simulink model "calibration_jacobian_n_8"  (R2018b)
settings: Solver=VariableStepAuto  StartTime=0.0  StopTime=10  RelTol=1e-3
values from neighbouring files (symbols this model uses):
  base_size = [0.2 0.3 1.5]    [robot_setup.m]    (also in robot_setup_delta_l.m)
  beam_length = 1.14    [robot_setup.m]    (also in robot_setup_delta_l.m)
  beam_radius = 0.032    [robot_setup.m]    (also in robot_setup_delta_l.m)
  fixture_height = 1.5    [robot_setup.m]    (also in robot_setup_delta_l.m)
  robot_frame_x = 0.15    [robot_setup.m]    (also in robot_setup_delta_l.m)
  T = 0.005    [robot_setup.m]    (also in robot_setup_delta_l.m)
  theta_m_des_calib = 0    [robot_setup_delta_l.m]
  wf_T_rf_left = [R_left, xyz_left'; 0 0 0 1]    [robot_setup.m]    (also in robot_setup_delta_l.m)
  wf_T_rf_right = [R_right, xyz_right'; 0 0 0 1]    [robot_setup.m]    (also in robot_setup_delta_l.m)
  xyz_0_rf_left = xyz_0_rf_left(1:3)    [robot_setup.m]    (also in robot_setup_delta_l.m)
  xyz_0_rf_right = xyz_0_rf_right(1:3)    [robot_setup.m]    (also in robot_setup_delta_l.m)
  yd_des_calib = 1    [robot_setup.m]    (also in robot_setup_delta_l.m = 0.9)
  ym_des_calib = 0    [robot_setup.m]    (also in robot_setup_delta_l.m)
  zd_des_calib = 0    [robot_setup.m]    (also in robot_setup_delta_l.m)
  zm_des_calib = 1.5    [robot_setup.m]    (also in robot_setup_delta_l.m)
undefined symbols (not defined in the file or in its folder): beam_wall, beam_width, Extr_Data_Box, Levenberg, Marquardt, num_elements, X, Y, Z
libraries: sm_lib x349, nesl_utility x63, sm_flex_body_lib x12, robotcorelib x4, simulink x2, robotmaniplib x2
(part 8 of 8)

== system calibration_jacobian_n_8/KUKA IIWA right/KUKA_iiwa 1 /iiwa_link_6 ==
  Inertia : sm_lib/Body Elements/Inertia  InertiaType=Custom  Mass=2.3466  MassUnits=kg  CenterOfMass=[0, 0, 0]  CenterOfMassUnits=m  MomentsOfInertia=[0.006509, 0.006259, 0.004527]  MomentsOfInertiaUnits=kg*m^2  ProductsOfInertia=[0.00031891, 0, 0]  ProductsOfInertiaUnits=kg*m^2  GraphicType=None  MarkerShape=Inertia  MarkerSize=20  GraphicVisPropType=SimpleVisualProperties  GraphicDiffuseColor=[0.5 0.5 0.5]  GraphicSpecularColor=[0.5 0.5 0.5 1.0]  GraphicAmbientColor=[0.15 0.15 0.15 1.0]  GraphicEmissiveColor=[0.0 0.0 0.0 1.0]  GraphicShininess=75  GraphicOpacity=1.0
  InertiaOriginTransform : sm_lib/Frames and Transforms/Rigid Transform  TranslationMethod=Cartesian  TranslationStandardOffset=0  TranslationLengthUnit=m  TranslationStandardAxis=+Z  TranslationCartesianOffset=[0, 0.0005999999999999999, 0.0004]  TranslationROffset=0  TranslationROffsetUnits=m  TranslationZOffset=0  TranslationZOffsetUnits=m  TranslationThetaOffset=0  TranslationThetaOffsetUnits=deg  RotationMethod=RotationSequence  RotationAngleUnits=deg  RotationStandardAxis=+Z  RotationAngle=0.0  RotationArbitraryAxis=[0 0 1]  FollAlignAxisA=+X  BaseAlignAxisA=+Y  FollAlignAxisB=+Y  BaseAlignAxisB=+Z  RotationSequenceAxes=BaseAxes  RotationSequence=XYZ  RotationSequenceAngles=[0, 0, 0]  RotationSequenceAnglesUnits=rad  RotationMatrix=[1 0 0; 0 1 0; 0 0 1]
  ReferenceFrame : sm_lib/Frames and Transforms/Reference Frame
  Visual : sm_lib/Body Elements/Solid  InertiaType=Custom  Mass=0  MassUnits=kg  CenterOfMass=[0, 0, 0]  CenterOfMassUnits=m  MomentsOfInertia=[0, 0, 0]  MomentsOfInertiaUnits=kg*m^2  ProductsOfInertia=[0, 0, 0]  ProductsOfInertiaUnits=kg*m^2  BasedOnType=Density  Density=1000  DensityUnits=kg/m^3  DoExposeReferenceFrame=on  SerializedFrames=<Frames/>  GraphicType=FromGeometry  MarkerShape=Sphere  MarkerSize=10  GraphicVisPropType=SimpleVisualProperties  GraphicDiffuseColor=[1, 0.423529411765, 0.0392156862745]  GraphicSpecularColor=[0.5 0.5 0.5 1.0]  GraphicAmbientColor=[0.15 0.15 0.15 1.0]  GraphicEmissiveColor=[0.0 0.0 0.0 1.0]  GraphicShininess=75  GraphicOpacity=1  GeometryShape=FromFile  RectangleSize=[1 1]  RectangleSizeUnits=m  BrickDimensions=[1 1 1]  BrickDimensionUnits=m  CylinderRadius=1  CylinderRadiusUnits=m  CylinderLength=1  CylinderLengthUnits=m  SphereRadius=1  SphereRadiusUnits=m  EllipsoidRadii=[1 1 1]  EllipsoidRadiiUnits=m  ExtrusionCrossSection=[1 1; -1 1; -1 -1; 1 -1]  ExtrusionCrossSectionUnits=m  ExtrusionLength=1  ExtrusionLengthUnits=m  PolygonNumSides=3  PolygonOuterRadius=1  PolygonOuterRadiusUnits=m  ExtGeomFileType=STL  ExtGeomFileName=iiwa_description/meshes/iiwa7/visual/link_6.stl  ExtGeomFileUnits=m  RevolutionCrossSection=[1 1; 1 -1; 2 -1; 2 1]  RevolutionCrossSectionUnits=m  RevolutionExtent=Full  RevolutionAngle=180  RevolutionAngleUnits=deg
  VisualOriginTransform : sm_lib/Frames and Transforms/Rigid Transform  TranslationMethod=Cartesian  TranslationStandardOffset=0  TranslationLengthUnit=m  TranslationStandardAxis=+Z  TranslationCartesianOffset=[0, 0, 0]  TranslationROffset=0  TranslationROffsetUnits=m  TranslationZOffset=0  TranslationZOffsetUnits=m  TranslationThetaOffset=0  TranslationThetaOffsetUnits=deg  RotationMethod=RotationSequence  RotationAngleUnits=deg  RotationStandardAxis=+Z  RotationAngle=0.0  RotationArbitraryAxis=[0 0 1]  FollAlignAxisA=+X  BaseAlignAxisA=+Y  FollAlignAxisB=+Y  BaseAlignAxisB=+Z  RotationSequenceAxes=BaseAxes  RotationSequence=XYZ  RotationSequenceAngles=[0, 0, 0]  RotationSequenceAnglesUnits=rad  RotationMatrix=[1 0 0; 0 1 0; 0 0 1]
  iiwa_joint_6_AxisInvTransform : sm_lib/Frames and Transforms/Rigid Transform  TranslationMethod=Cartesian  TranslationStandardOffset=0  TranslationLengthUnit=m  TranslationStandardAxis=+Z  TranslationCartesianOffset=[0, 0, 0]  TranslationROffset=0  TranslationROffsetUnits=m  TranslationZOffset=0  TranslationZOffsetUnits=m  TranslationThetaOffset=0  TranslationThetaOffsetUnits=deg  RotationMethod=ArbitraryAxis  RotationAngleUnits=rad  RotationStandardAxis=+Z  RotationAngle=0  RotationArbitraryAxis=[1, 0, 0]  FollAlignAxisA=+X  BaseAlignAxisA=+Y  FollAlignAxisB=+Y  BaseAlignAxisB=+Z  RotationSequenceAxes=FollowerAxes  RotationSequence=XYX  RotationSequenceAngles=[0 0 0]  RotationSequenceAnglesUnits=deg  RotationMatrix=[1 0 0; 0 1 0; 0 0 1]
  iiwa_joint_7_AxisTransform : sm_lib/Frames and Transforms/Rigid Transform  TranslationMethod=Cartesian  TranslationStandardOffset=0  TranslationLengthUnit=m  TranslationStandardAxis=+Z  TranslationCartesianOffset=[0, 0, 0]  TranslationROffset=0  TranslationROffsetUnits=m  TranslationZOffset=0  TranslationZOffsetUnits=m  TranslationThetaOffset=0  TranslationThetaOffsetUnits=deg  RotationMethod=ArbitraryAxis  RotationAngleUnits=rad  RotationStandardAxis=+Z  RotationAngle=0  RotationArbitraryAxis=[1, 0, 0]  FollAlignAxisA=+X  BaseAlignAxisA=+Y  FollAlignAxisB=+Y  BaseAlignAxisB=+Z  RotationSequenceAxes=FollowerAxes  RotationSequence=XYX  RotationSequenceAngles=[0 0 0]  RotationSequenceAnglesUnits=deg  RotationMatrix=[1 0 0; 0 1 0; 0 0 1]
  iiwa_joint_7_OriginTransform : sm_lib/Frames and Transforms/Rigid Transform  TranslationMethod=Cartesian  TranslationStandardOffset=0  TranslationLengthUnit=m  TranslationStandardAxis=+Z  TranslationCartesianOffset=[0, 0.081, 0.0607]  TranslationROffset=0  TranslationROffsetUnits=m  TranslationZOffset=0  TranslationZOffsetUnits=m  TranslationThetaOffset=0  TranslationThetaOffsetUnits=deg  RotationMethod=RotationSequence  RotationAngleUnits=deg  RotationStandardAxis=+Z  RotationAngle=0.0  RotationArbitraryAxis=[0 0 1]  FollAlignAxisA=+X  BaseAlignAxisA=+Y  FollAlignAxisB=+Y  BaseAlignAxisB=+Z  RotationSequenceAxes=BaseAxes  RotationSequence=XYZ  RotationSequenceAngles=[-1.57079632679, 3.14159265359, 0]  RotationSequenceAnglesUnits=rad  RotationMatrix=[1 0 0; 0 1 0; 0 0 1]
  F : PMIOPort  Side=Left
  F1 : PMIOPort  Port=2  Side=Right
  connections:
  Inertia/RConn1 -- InertiaOriginTransform/RConn1
  ReferenceFrame/RConn1 -- InertiaOriginTransform/LConn1 -- VisualOriginTransform/LConn1 -- iiwa_joint_6_AxisInvTransform/LConn1 -- iiwa_joint_7_OriginTransform/LConn1
  Visual/RConn1 -- VisualOriginTransform/RConn1
  iiwa_joint_6_AxisInvTransform/RConn1 -- F/RConn1
  iiwa_joint_7_AxisTransform/RConn1 -- F1/RConn1
  iiwa_joint_7_AxisTransform/LConn1 -- iiwa_joint_7_OriginTransform/RConn1

== system calibration_jacobian_n_8/KUKA IIWA right/KUKA_iiwa 1 /iiwa_link_7 ==
  Inertia : sm_lib/Body Elements/Inertia  InertiaType=Custom  Mass=3.129  MassUnits=kg  CenterOfMass=[0, 0, 0]  CenterOfMassUnits=m  MomentsOfInertia=[0.01464, 0.01465, 0.002872]  MomentsOfInertiaUnits=kg*m^2  ProductsOfInertia=[0, 0, 0.0005912]  ProductsOfInertiaUnits=kg*m^2  GraphicType=None  MarkerShape=Inertia  MarkerSize=20  GraphicVisPropType=SimpleVisualProperties  GraphicDiffuseColor=[0.5 0.5 0.5]  GraphicSpecularColor=[0.5 0.5 0.5 1.0]  GraphicAmbientColor=[0.15 0.15 0.15 1.0]  GraphicEmissiveColor=[0.0 0.0 0.0 1.0]  GraphicShininess=75  GraphicOpacity=1.0
  InertiaOriginTransform : sm_lib/Frames and Transforms/Rigid Transform  TranslationMethod=Cartesian  TranslationStandardOffset=0  TranslationLengthUnit=m  TranslationStandardAxis=+Z  TranslationCartesianOffset=[0, 0, 0.02]  TranslationROffset=0  TranslationROffsetUnits=m  TranslationZOffset=0  TranslationZOffsetUnits=m  TranslationThetaOffset=0  TranslationThetaOffsetUnits=deg  RotationMethod=RotationSequence  RotationAngleUnits=deg  RotationStandardAxis=+Z  RotationAngle=0.0  RotationArbitraryAxis=[0 0 1]  FollAlignAxisA=+X  BaseAlignAxisA=+Y  FollAlignAxisB=+Y  BaseAlignAxisB=+Z  RotationSequenceAxes=BaseAxes  RotationSequence=XYZ  RotationSequenceAngles=[0, 0, 0]  RotationSequenceAnglesUnits=rad  RotationMatrix=[1 0 0; 0 1 0; 0 0 1]
  ReferenceFrame : sm_lib/Frames and Transforms/Reference Frame
  Visual : sm_lib/Body Elements/Solid  InertiaType=Custom  Mass=0  MassUnits=kg  CenterOfMass=[0, 0, 0]  CenterOfMassUnits=m  MomentsOfInertia=[0, 0, 0]  MomentsOfInertiaUnits=kg*m^2  ProductsOfInertia=[0, 0, 0]  ProductsOfInertiaUnits=kg*m^2  BasedOnType=Density  Density=1000  DensityUnits=kg/m^3  DoExposeReferenceFrame=on  SerializedFrames=<Frames/>  GraphicType=FromGeometry  MarkerShape=Sphere  MarkerSize=10  GraphicVisPropType=SimpleVisualProperties  GraphicDiffuseColor=[0.4, 0.4, 0.4]  GraphicSpecularColor=[0.5 0.5 0.5 1.0]  GraphicAmbientColor=[0.15 0.15 0.15 1.0]  GraphicEmissiveColor=[0.0 0.0 0.0 1.0]  GraphicShininess=75  GraphicOpacity=1  GeometryShape=FromFile  RectangleSize=[1 1]  RectangleSizeUnits=m  BrickDimensions=[1 1 1]  BrickDimensionUnits=m  CylinderRadius=1  CylinderRadiusUnits=m  CylinderLength=1  CylinderLengthUnits=m  SphereRadius=1  SphereRadiusUnits=m  EllipsoidRadii=[1 1 1]  EllipsoidRadiiUnits=m  ExtrusionCrossSection=[1 1; -1 1; -1 -1; 1 -1]  ExtrusionCrossSectionUnits=m  ExtrusionLength=1  ExtrusionLengthUnits=m  PolygonNumSides=3  PolygonOuterRadius=1  PolygonOuterRadiusUnits=m  ExtGeomFileType=STL  ExtGeomFileName=iiwa_description/meshes/iiwa7/visual/link_7.stl  ExtGeomFileUnits=m  RevolutionCrossSection=[1 1; 1 -1; 2 -1; 2 1]  RevolutionCrossSectionUnits=m  RevolutionExtent=Full  RevolutionAngle=180  RevolutionAngleUnits=deg
  VisualOriginTransform : sm_lib/Frames and Transforms/Rigid Transform  TranslationMethod=Cartesian  TranslationStandardOffset=0  TranslationLengthUnit=m  TranslationStandardAxis=+Z  TranslationCartesianOffset=[0, 0, -0.0005]  TranslationROffset=0  TranslationROffsetUnits=m  TranslationZOffset=0  TranslationZOffsetUnits=m  TranslationThetaOffset=0  TranslationThetaOffsetUnits=deg  RotationMethod=RotationSequence  RotationAngleUnits=deg  RotationStandardAxis=+Z  RotationAngle=0.0  RotationArbitraryAxis=[0 0 1]  FollAlignAxisA=+X  BaseAlignAxisA=+Y  FollAlignAxisB=+Y  BaseAlignAxisB=+Z  RotationSequenceAxes=BaseAxes  RotationSequence=XYZ  RotationSequenceAngles=[0, 0, 0]  RotationSequenceAnglesUnits=rad  RotationMatrix=[1 0 0; 0 1 0; 0 0 1]
  iiwa_joint_7_AxisInvTransform : sm_lib/Frames and Transforms/Rigid Transform  TranslationMethod=Cartesian  TranslationStandardOffset=0  TranslationLengthUnit=m  TranslationStandardAxis=+Z  TranslationCartesianOffset=[0, 0, 0]  TranslationROffset=0  TranslationROffsetUnits=m  TranslationZOffset=0  TranslationZOffsetUnits=m  TranslationThetaOffset=0  TranslationThetaOffsetUnits=deg  RotationMethod=ArbitraryAxis  RotationAngleUnits=rad  RotationStandardAxis=+Z  RotationAngle=0  RotationArbitraryAxis=[1, 0, 0]  FollAlignAxisA=+X  BaseAlignAxisA=+Y  FollAlignAxisB=+Y  BaseAlignAxisB=+Z  RotationSequenceAxes=FollowerAxes  RotationSequence=XYX  RotationSequenceAngles=[0 0 0]  RotationSequenceAnglesUnits=deg  RotationMatrix=[1 0 0; 0 1 0; 0 0 1]
  iiwa_joint_ee_OriginTransform : sm_lib/Frames and Transforms/Rigid Transform  TranslationMethod=Cartesian  TranslationStandardOffset=0  TranslationLengthUnit=m  TranslationStandardAxis=+Z  TranslationCartesianOffset=[0, 0, 0.045]  TranslationROffset=0  TranslationROffsetUnits=m  TranslationZOffset=0  TranslationZOffsetUnits=m  TranslationThetaOffset=0  TranslationThetaOffsetUnits=deg  RotationMethod=RotationSequence  RotationAngleUnits=deg  RotationStandardAxis=+Z  RotationAngle=0.0  RotationArbitraryAxis=[0 0 1]  FollAlignAxisA=+X  BaseAlignAxisA=+Y  FollAlignAxisB=+Y  BaseAlignAxisB=+Z  RotationSequenceAxes=BaseAxes  RotationSequence=XYZ  RotationSequenceAngles=[0, -1.57079632679, 0]  RotationSequenceAnglesUnits=rad  RotationMatrix=[1 0 0; 0 1 0; 0 0 1]
  iiwa_joint_ee_kuka_OriginTransform : sm_lib/Frames and Transforms/Rigid Transform  TranslationMethod=Cartesian  TranslationStandardOffset=0  TranslationLengthUnit=m  TranslationStandardAxis=+Z  TranslationCartesianOffset=[0, 0, 0.045]  TranslationROffset=0  TranslationROffsetUnits=m  TranslationZOffset=0  TranslationZOffsetUnits=m  TranslationThetaOffset=0  TranslationThetaOffsetUnits=deg  RotationMethod=RotationSequence  RotationAngleUnits=deg  RotationStandardAxis=+Z  RotationAngle=0.0  RotationArbitraryAxis=[0 0 1]  FollAlignAxisA=+X  BaseAlignAxisA=+Y  FollAlignAxisB=+Y  BaseAlignAxisB=+Z  RotationSequenceAxes=BaseAxes  RotationSequence=XYZ  RotationSequenceAngles=[3.14159265359, 3.14159265359, 3.14159265359]  RotationSequenceAnglesUnits=rad  RotationMatrix=[1 0 0; 0 1 0; 0 0 1]
  F : PMIOPort  Side=Left
  F2 : PMIOPort  Port=2  Side=Right
  F1 : PMIOPort  Port=3  Side=Right
  connections:
  Inertia/RConn1 -- InertiaOriginTransform/RConn1
  ReferenceFrame/RConn1 -- InertiaOriginTransform/LConn1 -- iiwa_joint_ee_OriginTransform/LConn1 -- iiwa_joint_ee_kuka_OriginTransform/LConn1 -- iiwa_joint_7_AxisInvTransform/LConn1 -- VisualOriginTransform/LConn1
  Visual/RConn1 -- VisualOriginTransform/RConn1
  iiwa_joint_7_AxisInvTransform/RConn1 -- F/RConn1
  iiwa_joint_ee_OriginTransform/RConn1 -- F1/RConn1
  iiwa_joint_ee_kuka_OriginTransform/RConn1 -- F2/RConn1

== system calibration_jacobian_n_8/KUKA IIWA right/KUKA_iiwa 1 /iiwa_link_ee_weld ==
  ReferenceFrame : sm_lib/Frames and Transforms/Reference Frame
  F : PMIOPort  Side=Left
  connections:
  ReferenceFrame/RConn1 -- F/RConn1

== system calibration_jacobian_n_8/KUKA IIWA right/KUKA_iiwa 1 /world ==
  ReferenceFrame : sm_lib/Frames and Transforms/Reference Frame
  world_iiwa_joint_OriginTransform : sm_lib/Frames and Transforms/Rigid Transform  TranslationMethod=Cartesian  TranslationStandardOffset=0  TranslationLengthUnit=m  TranslationStandardAxis=+Z  TranslationCartesianOffset=base_pos  TranslationROffset=0  TranslationROffsetUnits=m  TranslationZOffset=0  TranslationZOffsetUnits=m  TranslationThetaOffset=0  TranslationThetaOffsetUnits=deg  RotationMethod=RotationSequence  RotationAngleUnits=deg  RotationStandardAxis=+Z  RotationAngle=0.0  RotationArbitraryAxis=[0 0 1]  FollAlignAxisA=+X  BaseAlignAxisA=+Y  FollAlignAxisB=+Y  BaseAlignAxisB=+Z  RotationSequenceAxes=BaseAxes  RotationSequence=ZYX  RotationSequenceAngles=base_rot  RotationSequenceAnglesUnits=rad  RotationMatrix=[1 0 0; 0 1 0; 0 0 1]
  F : PMIOPort  Side=Left
  F1 : PMIOPort  Port=2  Side=Right
  connections:
  world_iiwa_joint_OriginTransform/LConn1 -- ReferenceFrame/RConn1 -- F/RConn1
  world_iiwa_joint_OriginTransform/RConn1 -- F1/RConn1

== matlab function calibration_jacobian_n_8/CONTROLLER/Controller ==
  data: T input; xyz_beam_wf_des input; xyz_rf_new output; wf_T_rf_left input; wf_T_rf_right input; ypr_rf_old input; xyz_rf_old input; trigger_old input; ypr_rf_new output; beam_measured_input output; trigger_new output
function [xyz_rf_new, ypr_rf_new, beam_measured_input, trigger_new]   = robot_ctrl(T, xyz_beam_wf_des, wf_T_rf_left, wf_T_rf_right, ypr_rf_old, xyz_rf_old, trigger_old)

    thresh_l = 10^-3;
    delta_trasl = 0.2;
    
    delta_l = 0.05;
    delta_rot = pi/16;
    
    trigger_new = trigger_old;
    
    ypr_rf_new_left = ypr_rf_old(1:3);
    ypr_rf_new_right = ypr_rf_old(4:6);
   
    xyz_rf_new_left = xyz_rf_old(1:3);
    xyz_rf_new_right = xyz_rf_old(4:6);
    
     % work in the world frame
    xyz_wf_new_left = wf_T_rf_left * [xyz_rf_new_left;1];
    xyz_wf_new_right = wf_T_rf_right * [xyz_rf_new_right;1];    

    yd_wf_des = xyz_beam_wf_des(1);
    ym_wf_des = xyz_beam_wf_des(2);
    zd_wf_des = xyz_beam_wf_des(3);
    zm_wf_des = xyz_beam_wf_des(4);
    
    theta_m_wf_des = xyz_beam_wf_des(5);
    
    y_wf_new_left = xyz_wf_new_left(2);
    y_wf_new_right = xyz_wf_new_right(2);
    z_wf_new_left = xyz_wf_new_left(3);
    z_wf_new_right = xyz_wf_new_right(3);
    
    yd_wf = y_wf_new_left-y_wf_new_right;
    ym_wf = (y_wf_new_left+y_wf_new_right)/2;
    zd_wf = (z_wf_new_left-z_wf_new_right);
    zm_wf = (z_wf_new_left+z_wf_new_right)/2;
    
    
    d = sqrt( yd_wf_des^2 + zd_wf_des^2 );
    yd_theta_wf_des = d*cos(theta_m_wf_des);
    zd_theta_wf_des = d*sin(theta_m_wf_des);
    yd_theta_wf_des_p = d*cos(theta_m_wf_des+delta_rot);
    zd_theta_wf_des_p = d*sin(theta_m_wf_des+delta_rot);
    yd_theta_wf_des_m = d*cos(theta_m_wf_des-delta_rot);
    zd_theta_wf_des_m = d*sin(theta_m_wf_des-delta_rot);
    
    theta_m_wf = atan2(zd_wf, yd_wf);
    
    cond_yd = abs(yd_wf_des-yd_wf) < thresh_l;
    cond_yd_p = abs(yd_wf_des+delta_l-yd_wf) < thresh_l && trigger_new(1,1)==1 && trigger_new(1,2) == 0;
    cond_yd_m = abs(yd_wf_des-delta_l-yd_wf) < thresh_l && trigger_new(1,2)==1 && trigger_new(1,3) == 0;
    
    cond_ym = abs(ym_wf_des-ym_wf) < thresh_l;
    cond_ym_p = abs(ym_wf_des+delta_l-ym_wf) < thresh_l && trigger_new(2,1) == 1;
    cond_ym_m = abs(ym_wf_des-delta_l-ym_wf) < thresh_l && trigger_new(2,2) == 1;
    
    cond_zd = abs(zd_wf_des-zd_wf) < thresh_l;
    cond_zd_p = abs(zd_wf_des+delta_l-zd_wf) < thresh_l && trigger_new(3,1)==1 && trigger_new(3,2) == 0;
    cond_zd_m = abs(zd_wf_des-delta_l-zd_wf) < thresh_l && trigger_new(3,2)==1 && trigger_new(3,3) == 0;
    
    cond_zm = abs(zm_wf_des-zm_wf) < thresh_l;
    cond_zm_p = abs(zm_wf_des+delta_l-zm_wf) < thresh_l && trigger_new(4,1)==1;
    cond_zm_m = abs(zm_wf_des-delta_l-zm_wf) < thresh_l && trigger_new(4,2)==1;
    
    cond_theta_m = abs(yd_theta_wf_des-yd_wf) < 3*thresh_l && abs(zd_theta_wf_des-zd_wf) < 3*thresh_l;
    cond_theta_m_p = abs(yd_theta_wf_des_p-yd_wf) < 3*thresh_l && abs(zd_theta_wf_des_p-zd_wf) < 3*thresh_l && trigger_new(5,1)==1 && trigger_new(5,2) == 0; 
    cond_theta_m_m = abs(yd_theta_wf_des_m-yd_wf) < 3*thresh_l && abs(zd_theta_wf_des_m-zd_wf) < 3*thresh_l && trigger_new(5,2)==1 && trigger_new(5,3) == 0;
             
    
    %% relative distance along y (wf)
    if cond_yd
        trigger_new(1,1) = 1;
    end
    if cond_yd_p 
        trigger_new(1,2) = 1;
        trigger_new(1,1) = 0;
    end
    if cond_yd_m 
        trigger_new(1,3) = 1;
        trigger_new(1,1) = 0;
    end   
        %% absolute distance from origin
    if cond_ym 
        trigger_new(2,1) = 1;
    end
    if cond_ym_p
        trigger_new(2,2) = 1;
        trigger_new(2,1) = 0;
    end
    if cond_ym_m
        trigger_new(2,3) = 1;
        trigger_new(2,1) = 0;
    end
    
    %% relative distance along z (wf)
    if cond_zd
        trigger_new(3,1) = 1;
    end
    if cond_zd_p && trigger_new(4,3) == 0
        trigger_new(3,2) = 1;
        trigger_new(3,1) = 0;
    end
    if cond_zd_m && trigger_new(4,3) == 0
        trigger_new(3,3) = 1;
        trigger_new(3,1) = 0;
    end   
    
    %% absolute distance along z (wf)
    if cond_zm
        trigger_new(4,1) = 1;
    end
    if cond_zm_p 
        trigger_new(4,2) = 1;
        trigger_new(4,1) = 0;
    end
    if cond_zm_m 
        trigger_new(4,3) = 1;
        trigger_new(4,1) = 0;
    end   
    
    %% absolute orientation around x (wf)
    if cond_theta_m
        trigger_new(5,1) = 1;
    end
    if cond_theta_m_p && trigger_new(4,3) == 1
        trigger_new(5,2) = 1;
        trigger_new(5,1) = 0;
    end
    if cond_theta_m_m && trigger_new(4,3) == 1
        trigger_new(5,3) = 1;
        trigger_new(5,1) = 0;
    end  
    
    y_d = [-9999,-9999];
    y_m = [-9999,-9999];
    z_d = [-9999,-9999];
    z_m = [-9999,-9999];
    theta_m = [-9999,-9999];
    
    %% relative distance along y (wf)
    if ~cond_yd && trigger_new(1,1) == 0
  
        [xyz_wf_new_left(2), xyz_wf_new_right(2)] = symmetric_pos_ctrl(yd_wf, yd_wf_des, delta_trasl, T, -1, xyz_wf_new_left(2), xyz_wf_new_right(2));
    
    elseif ~cond_yd_p && trigger_new(1,2) == 0
        
        y_d = [yd_wf, -9999];
        [xyz_wf_new_left(2), xyz_wf_new_right(2)] = symmetric_pos_ctrl(yd_wf, yd_wf_des+delta_l, delta_trasl, T, -1, xyz_wf_new_left(2), xyz_wf_new_right(2));
    
    elseif ~cond_yd_m && trigger_new(1,3) == 0
        
        y_d = [-9999, yd_wf];
        [xyz_wf_new_left(2), xyz_wf_new_right(2)] = symmetric_pos_ctrl(yd_wf, yd_wf_des-delta_l, delta_trasl, T, -1, xyz_wf_new_left(2), xyz_wf_new_right(2));
    %% absolute distance along y (wf)
    elseif ~cond_ym && trigger_new(2,1)==0
              
        [xyz_wf_new_left(2), xyz_wf_new_right(2)] = symmetric_pos_ctrl(ym_wf, ym_wf_des, delta_trasl, T, 1, xyz_wf_new_left(2), xyz_wf_new_right(2));
        
    elseif ~cond_ym_p && trigger_new(2,2)==0
        
        y_m = [ym_wf, -9999];
        [xyz_wf_new_left(2), xyz_wf_new_right(2)] = symmetric_pos_ctrl(ym_wf, ym_wf_des+delta_l, delta_trasl, T, 1, xyz_wf_new_left(2), xyz_wf_new_right(2));
        
    elseif ~cond_ym_m && trigger_new(2,3)==0
        
        y_m = [-9999, ym_wf];
        [xyz_wf_new_left(2), xyz_wf_new_right(2)] = symmetric_pos_ctrl(ym_wf, ym_wf_des-delta_l, delta_trasl, T, 1, xyz_wf_new_left(2), xyz_wf_new_right(2));
   
    %% relative distance along z (wf)
    elseif ~cond_zd && trigger_new(3,1) == 0
  
        [xyz_wf_new_left(3), xyz_wf_new_right(3)] = symmetric_pos_ctrl(zd_wf, zd_wf_des, delta_trasl, T, -1, xyz_wf_new_left(3), xyz_wf_new_right(3));
    
    elseif ~cond_zd_p && trigger_new(3,2) == 0
        
        z_d = [zd_wf, -9999];
        [xyz_wf_new_left(3), xyz_wf_new_right(3)] = symmetric_pos_ctrl(zd_wf, zd_wf_des+delta_l, delta_trasl, T, -1, xyz_wf_new_left(3), xyz_wf_new_right(3));
    
    elseif ~cond_zd_m && trigger_new(3,3) == 0
        
        z_d = [-9999, zd_wf];
        [xyz_wf_new_left(3), xyz_wf_new_right(3)] = symmetric_pos_ctrl(zd_wf,  zd_wf_des-delta_l, delta_trasl, T, -1, xyz_wf_new_left(3), xyz_wf_new_right(3));

 %% absolute distance along z (wf)
    elseif ~cond_zm && trigger_new(4,1) == 0
  
        [xyz_wf_new_left(3), xyz_wf_new_right(3)] = symmetric_pos_ctrl(zm_wf, zm_wf_des, delta_trasl, T, 1, xyz_wf_new_left(3), xyz_wf_new_right(3));
    
    elseif ~cond_zm_p && trigger_new(4,2) == 0
        
        z_m = [zm_wf, -9999];
        [xyz_wf_new_left(3), xyz_wf_new_right(3)] = symmetric_pos_ctrl(zm_wf, zm_wf_des+delta_l, delta_trasl, T, 1, xyz_wf_new_left(3), xyz_wf_new_right(3));
    
    elseif ~cond_zm_m && trigger_new(4,3) == 0
        
        z_m = [-9999, zm_wf];
        [xyz_wf_new_left(3), xyz_wf_new_right(3)] = symmetric_pos_ctrl(zm_wf,  zm_wf_des-delta_l, delta_trasl, T, 1, xyz_wf_new_left(3), xyz_wf_new_right(3));
    %% absolute orientation around z (wf)    
%      elseif ~cond_theta_m && trigger_new(5,1) == 0
%  
%         [xyz_wf_new_left(2), xyz_wf_new_right(2)] = symmetric_pos_ctrl(yd_wf, yd_theta_wf_des, 1.5*delta_trasl*cos(theta_m_wf_des+delta_rot), T, -1, xyz_wf_new_left(2), xyz_wf_new_right(2));
%         [xyz_wf_new_left(3), xyz_wf_new_right(3)] = symmetric_pos_ctrl(zd_wf, zd_theta_wf_des, 1.5*delta_trasl*sin(theta_m_wf_des+delta_rot), T, -1, xyz_wf_new_left(3), xyz_wf_new_right(3));
% 
%      elseif ~cond_theta_m_p && trigger_new(5,2) == 0
%          
%         theta_m = [theta_m_wf, -9999];
%         [xyz_wf_new_left(2), xyz_wf_new_right(2)] = symmetric_pos_ctrl(yd_wf, yd_theta_wf_des_p, 1.5*delta_trasl*cos(theta_m_wf_des+delta_rot), T, -1, xyz_wf_new_left(2), xyz_wf_new_right(2));
%         [xyz_wf_new_left(3), xyz_wf_new_right(3)] = symmetric_pos_ctrl(zd_wf, zd_theta_wf_des_p, 1.5*delta_trasl*sin(theta_m_wf_des+delta_rot), T, -1, xyz_wf_new_left(3), xyz_wf_new_right(3));
%      
%     elseif ~cond_theta_m_m && trigger_new(5,3) == 0
%         
%         theta_m = [-9999, theta_m_wf];
%         [xyz_wf_new_left(2), xyz_wf_new_right(2)] = symmetric_pos_ctrl(yd_wf, yd_theta_wf_des_m, 1.5*delta_trasl*cos(theta_m_wf_des+delta_rot), T, -1, xyz_wf_new_left(2), xyz_wf_new_right(2));
%         [xyz_wf_new_left(3), xyz_wf_new_right(3)] = symmetric_pos_ctrl(zd_wf, zd_theta_wf_des_m, 1.5*delta_trasl*sin(theta_m_wf_des+delta_rot), T, -1, xyz_wf_new_left(3), xyz_wf_new_right(3));
     end
    
    beam_measured_input = [y_d, y_m, z_d, z_m, theta_m];
    
    xyz_rf_new_left = (wf_T_rf_left^-1)*xyz_wf_new_left;
    xyz_rf_new_right = (wf_T_rf_right^-1)*xyz_wf_new_right;
    
    ypr_rf_new = [ypr_rf_new_left;ypr_rf_new_right];
    xyz_rf_new = [xyz_rf_new_left(1:3);xyz_rf_new_right(1:3)];
    
    
    
    

end
